simulink model "transformline"  (R2023b)
settings: Solver=VariableStepAuto  StartTime=0.0  StopTime=1e-6  RelTol=1e-3
libraries: fl_lib x24, XerolySkinner x2
settings Model: Creator=XerolySkinner  LastModifiedBy=XerolySkinner

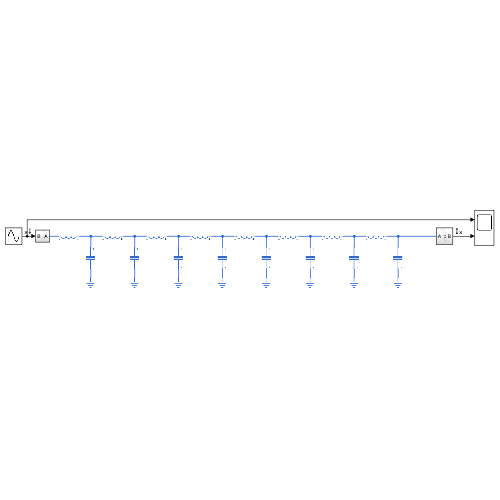
[thumbnail: Simulink's stored preview of the top-level diagram]
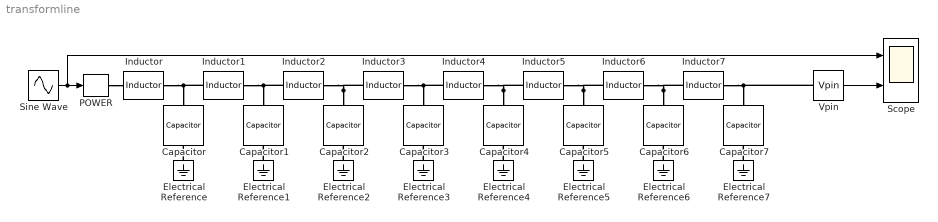
== system transformline ==
  Capacitor{,1..7} (8 alike) : fl_lib/Electrical/Electrical Elements/Capacitor  c=500e-15 F  r=1e-6 Ohm  g=0 1/Ohm  i_specify=off  i_priority=None  i=0 A  i_nominal_specify=off  i_nominal_unit=A  i_nominal_value=1  v_specify=off  v_priority=None  v=0 V  v_nominal_specify=off  v_nominal_unit=V  v_nominal_value=1  vc_specify=off  vc_priority=High  vc=0 V  vc_nominal_specify=off  vc_nominal_unit=V  vc_nominal_value=1
  Electrical Reference{,1..7} (8 alike) : fl_lib/Electrical/Electrical Elements/Electrical Reference
  Inductor{,1..7} (8 alike) : fl_lib/Electrical/Electrical Elements/Inductor  l=1.25e-9 H  r=0 Ohm  g=1e-9 1/Ohm  i_specify=off  i_priority=None  i=0 A  i_nominal_specify=off  i_nominal_unit=A  i_nominal_value=1  v_specify=off  v_priority=None  v=0 V  v_nominal_specify=off  v_nominal_unit=V  v_nominal_value=1  i_L_specify=off  i_L_priority=High  i_L=0 A  i_L_nominal_specify=off  i_L_nominal_unit=A  i_L_nominal_value=1
  POWER : XerolySkinner/POWER  SystemSampleTime=-1  VariantActivationTime=update diagram  AllowFlexibleInterface=on  Latency=0  AutoFrameSizeCalculation=off
      settings: SourceProductName=XerolySkinner
  Scope : Scope  NumInputPorts=2
  Sine Wave : Sin  Frequency=1/7e9  SampleTime=0
  Vpin : XerolySkinner/Vpin  SystemSampleTime=-1  VariantActivationTime=update diagram  AllowFlexibleInterface=on  Latency=0  AutoFrameSizeCalculation=off
      settings: SourceProductName=XerolySkinner
  wires:
  Vpin/1 -> Scope/2
  Sine Wave/1 -> Scope/1, POWER/1
  connections:
  Inductor/LConn1 -- Inductor1/RConn1 -- Capacitor/LConn1
  Electrical Reference/LConn1 -- Capacitor/RConn1
  Electrical Reference1/LConn1 -- Capacitor1/RConn1
  Inductor1/LConn1 -- Inductor2/RConn1 -- Capacitor1/LConn1
  Capacitor2/LConn1 -- Inductor2/LConn1 -- Inductor3/RConn1
  Electrical Reference3/LConn1 -- Capacitor3/RConn1
  Electrical Reference2/LConn1 -- Capacitor2/RConn1
  Inductor3/LConn1 -- Inductor4/RConn1 -- Capacitor3/LConn1
  Capacitor4/LConn1 -- Inductor4/LConn1 -- Inductor5/RConn1
  Capacitor6/LConn1 -- Inductor6/LConn1 -- Inductor7/RConn1
  Capacitor5/LConn1 -- Inductor5/LConn1 -- Inductor6/RConn1
  Inductor7/LConn1 -- Vpin/LConn1 -- Capacitor7/LConn1
  Electrical Reference6/LConn1 -- Capacitor6/RConn1
  Electrical Reference4/LConn1 -- Capacitor4/RConn1
  Electrical Reference7/LConn1 -- Capacitor7/RConn1
  Electrical Reference5/LConn1 -- Capacitor5/RConn1
  POWER/RConn1 -- Inductor/RConn1
